simulink model "singlesource"  (Simulink 8.4)
settings: Solver=ode23tb  StartTime=0.0  StopTime=1  MaxStep=0.01  RelTol=1e-3
undefined symbols (not defined in the file): sigbuilder_block
libraries: powerlib x135, simulink x25, dsparch4 x2, powerlib_meascontrol x1
(part 1 of 2)
settings Model: Creator=Muruganandham  LastModifiedBy=SELVA
settings SolverCC: ZeroCrossControl=DisableAll

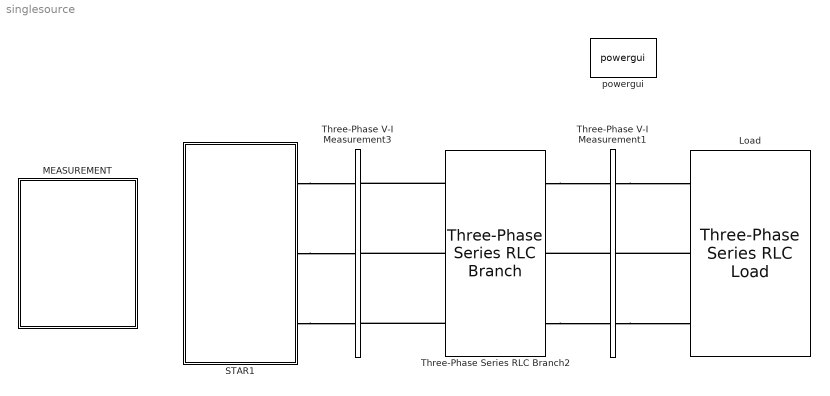
== system singlesource ==
  " Load" : powerlib/Elements/Three-Phase Series RLC Load  LConnTagsString=A|B|C  Configuration=Y (grounded)  NominalVoltage=410  NominalFrequency=50  ActivePower=5e3  InductivePower=0  CapacitivePower=0  Measurements=None  LoadType=constant Z
  MEASUREMENT : Subsystem
  STAR1 : Subsystem
  Three-Phase Series RLC Branch2 : powerlib/Elements/Three-Phase Series RLC Branch  LConnTagsString=A|B|C  RConnTagsString=A|B|C  BranchType=L  Resistance=0.0000001  Inductance=30e-3  Capacitance=3.5e-6  Measurements=None
  Three-Phase V-I Measurement1 : powerlib/Measurements/Three-Phase V-I Measurement  VoltageMeasurement=phase-to-phase  SetLabelV=on  LabelV=Vabc1  Vpu=off  VpuLL=off  CurrentMeasurement=yes  SetLabelI=on  LabelI=Iabc1  Ipu=off  Pbase=100e6  Vbase=500e3  OutputType=Complex  PhasorSimulation=off  PSBequivalent=0
  Three-Phase V-I Measurement3 : powerlib/Measurements/Three-Phase V-I Measurement  VoltageMeasurement=phase-to-phase  SetLabelV=on  LabelV=Vabc  Vpu=off  VpuLL=off  CurrentMeasurement=yes  SetLabelI=on  LabelI=Iabc  Ipu=off  Pbase=100e6  Vbase=500e3  OutputType=Complex  PhasorSimulation=off  PSBequivalent=0
  powergui : powerlib/powergui  Priority=1  SimulationMode=Discrete  SolverType=Tustin/Backward Euler (TBE)  SampleTime=5e-6  frequency=60  SPID=off  DisableSnubberDevices=off  DisableRonSwitches=off  DisableVfSwitches=off  SwTol=0  DisplayEquations=off  Interpol=off  methode=off  Ts=0  frequencyindice=0  Pbase=100e6  ErrMax=1e-4  Iterations=50  UnitsV=kV  UnitsW=MW  FunctionMessages=off  echomessages=off  HookPort=off  EnableUseOfTLC=off  x0status=blocks  RestoreLinks=warning  ResistiveCurrentMeasurement=off  Frange=[0:2:500]  Ylog=off  Xlog=on  ShowGrid=off  save=off  variable=ZData  structure=bn4  ZoomFFT=off  StartTime=0.5  cycles=1  DisplayStyle=1  fundamental=50  FreqAxis=off  MaxFrequency=1000  frequencyindicesteady=1  RmsSteady=1  display=off
  connections:
  Three-Phase V-I Measurement1/LConn1 -- " Load"/LConn1
  " Load"/LConn2 -- Three-Phase V-I Measurement1/LConn2
  Three-Phase V-I Measurement1/LConn3 -- " Load"/LConn3
  STAR1/RConn1 -- Three-Phase V-I Measurement3/RConn1
  STAR1/RConn2 -- Three-Phase V-I Measurement3/RConn2
  STAR1/RConn3 -- Three-Phase V-I Measurement3/RConn3
  Three-Phase Series RLC Branch2/LConn2 -- Three-Phase V-I Measurement3/LConn2
  Three-Phase Series RLC Branch2/LConn1 -- Three-Phase V-I Measurement3/LConn1
  Three-Phase Series RLC Branch2/LConn3 -- Three-Phase V-I Measurement3/LConn3
  Three-Phase Series RLC Branch2/RConn1 -- Three-Phase V-I Measurement1/RConn1
  Three-Phase Series RLC Branch2/RConn3 -- Three-Phase V-I Measurement1/RConn3
  Three-Phase V-I Measurement1/RConn2 -- Three-Phase Series RLC Branch2/RConn2

== system singlesource/MEASUREMENT ==
  Analog Filter Design : dsparch4/Analog Filter Design  method=Butterworth  filttype=Lowpass  N=8  Wlo=30  Whi=80  Rp=2  Rs=40
  Analog Filter Design1 : dsparch4/Analog Filter Design  method=Butterworth  filttype=Lowpass  N=8  Wlo=30  Whi=80  Rp=2  Rs=40
  Mux3 : Mux  Inputs=2
  "Power (3ph, Instantaneous)" : powerlib_meascontrol/Measurements/Power (3ph, Instantaneous)
  Scope{1,3,8..9} (4 alike) : Scope
      Scope1 settings: TimeRange=0.5  YMin=-800  YMax=800  SaveName=bn3
      Scope3 settings: TimeRange=0.5  YMin=-1000  YMax=6000  SaveName=bn2
      Scope8 settings: TimeRange=0.5  YMin=-600  YMax=800  SaveName=bn4
      Scope9 settings: YMin=-20  YMax=20
  wires:
  [Vabc] -> Scope1/1
  [Vabc1] -> "Power (3ph, Instantaneous)"/1, Scope8/1
  [Iabc1] -> "Power (3ph, Instantaneous)"/2, Scope9/1
  "Power (3ph, Instantaneous)"/1 -> Analog Filter Design/1
  "Power (3ph, Instantaneous)"/2 -> Analog Filter Design1/1
  Mux3/1 -> Scope3/1
  Analog Filter Design/1 -> Mux3/1
  Analog Filter Design1/1 -> Mux3/2

== system singlesource/STAR1 ==
  "B " : Subsystem
  DC : Subsystem
  DC1 : Subsystem
  DC2 : Subsystem
  Ground : powerlib/Elements/Ground  LConnTagsString=a
  PULSE : Subsystem  mask{fc=1000, m=1, d=0.0067}
      mask prompts: fc "Switching Frequency"; m "Modulation Index"; d "Delay"
  R : Subsystem
  Y : Subsystem
  A : PMIOPort  Tag=PMCPort  Port=1  Side=Right
  B : PMIOPort  Tag=PMCPort  Port=2  Side=Right
  C : PMIOPort  Tag=PMCPort  Port=3  Side=Right
  connections:
  Y/RConn2 -- Ground/LConn1 -- "B "/RConn2 -- R/RConn2
  DC/RConn1 -- R/LConn1
  DC/RConn3 -- R/LConn3
  DC/RConn4 -- R/LConn4
  DC/RConn9 -- R/LConn9
  DC/RConn2 -- R/LConn2
  DC/RConn5 -- R/LConn5
  DC/RConn7 -- R/LConn7
  DC/RConn6 -- R/LConn6
  DC/RConn8 -- R/LConn8
  DC/RConn10 -- R/LConn10
  DC1/RConn1 -- Y/LConn1
  DC1/RConn2 -- Y/LConn2
  DC1/RConn3 -- Y/LConn3
  DC1/RConn4 -- Y/LConn4
  DC1/RConn5 -- Y/LConn5
  DC1/RConn6 -- Y/LConn6
  DC1/RConn7 -- Y/LConn7
  DC1/RConn8 -- Y/LConn8
  DC1/RConn9 -- Y/LConn9
  DC1/RConn10 -- Y/LConn10
  DC2/RConn1 -- "B "/LConn1
  DC2/RConn2 -- "B "/LConn2
  DC2/RConn3 -- "B "/LConn3
  DC2/RConn4 -- "B "/LConn4
  DC2/RConn5 -- "B "/LConn5
  DC2/RConn6 -- "B "/LConn6
  DC2/RConn7 -- "B "/LConn7
  DC2/RConn8 -- "B "/LConn8
  DC2/RConn9 -- "B "/LConn9
  DC2/RConn10 -- "B "/LConn10
  A/RConn1 -- R/RConn1
  B/RConn1 -- Y/RConn1
  C/RConn1 -- "B "/RConn1

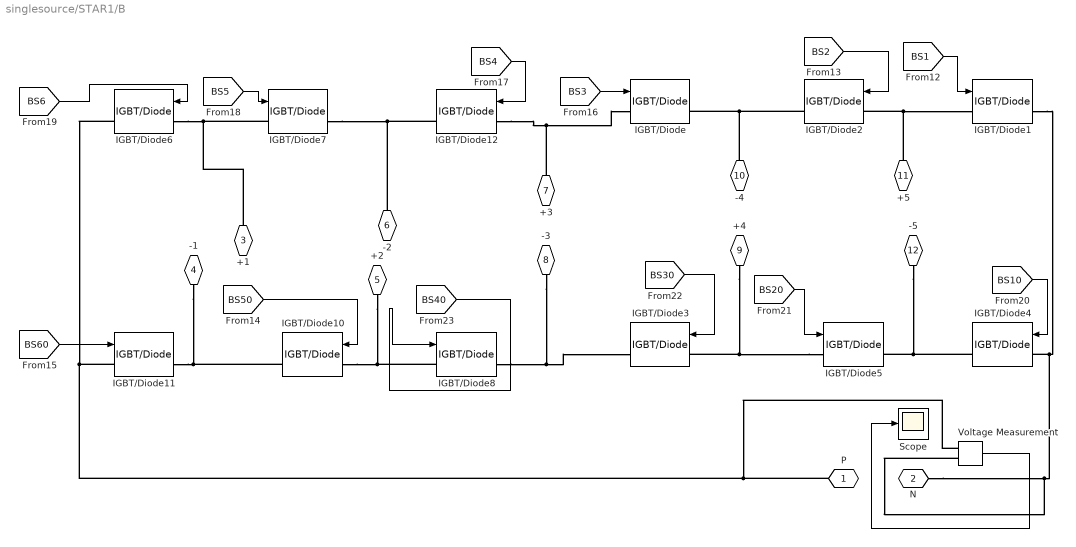
== system singlesource/STAR1/B  ==
  IGBT/Diode{,1..8,10..12} (12 alike) : powerlib/Power Electronics/IGBT//Diode  Ron=1e-3  Rs=1e5  Cs=inf  Measurements=on
  Scope : Scope
  Voltage Measurement : powerlib/Measurements/Voltage Measurement  PhasorSimulation=off  OutputType=Complex  PSBequivalent=0
  P : PMIOPort  Tag=PMCPort  Port=1  Side=Right
  N : PMIOPort  Tag=PMCPort  Port=2  Side=Right
  +1 : PMIOPort  Tag=PMCPort  Port=3  Side=Left
  -1 : PMIOPort  Tag=PMCPort  Port=4  Side=Left
  +2 : PMIOPort  Tag=PMCPort  Port=5  Side=Left
  -2 : PMIOPort  Tag=PMCPort  Port=6  Side=Left
  +3 : PMIOPort  Tag=PMCPort  Port=7  Side=Left
  -3 : PMIOPort  Tag=PMCPort  Port=8  Side=Left
  +4 : PMIOPort  Tag=PMCPort  Port=9  Side=Left
  -4 : PMIOPort  Tag=PMCPort  Port=10  Side=Left
  +5 : PMIOPort  Tag=PMCPort  Port=11  Side=Left
  -5 : PMIOPort  Tag=PMCPort  Port=12  Side=Left
  wires:
  [BS10] -> IGBT/Diode4/1
  [BS2] -> IGBT/Diode2/1
  [BS20] -> IGBT/Diode5/1
  [BS3] -> IGBT/Diode/1
  [BS30] -> IGBT/Diode3/1
  [BS40] -> IGBT/Diode8/1
  [BS6] -> IGBT/Diode6/1
  [BS4] -> IGBT/Diode12/1
  [BS5] -> IGBT/Diode7/1
  [BS50] -> IGBT/Diode10/1
  [BS60] -> IGBT/Diode11/1
  Voltage Measurement/1 -> Scope/1
  [BS1] -> IGBT/Diode1/1
  connections:
  IGBT/Diode2/RConn1 -- -4/RConn1 -- IGBT/Diode/RConn1
  IGBT/Diode2/LConn1 -- IGBT/Diode1/LConn1 -- +5/RConn1
  IGBT/Diode5/LConn1 -- +4/RConn1 -- IGBT/Diode3/LConn1
  IGBT/Diode4/RConn1 -- -5/RConn1 -- IGBT/Diode5/RConn1
  IGBT/Diode4/LConn1 -- IGBT/Diode1/RConn1 -- N/RConn1 -- Voltage Measurement/LConn2
  IGBT/Diode7/LConn1 -- +1/RConn1 -- IGBT/Diode6/LConn1
  IGBT/Diode12/RConn1 -- IGBT/Diode7/RConn1 -- -2/RConn1
  IGBT/Diode10/RConn1 -- IGBT/Diode11/RConn1 -- -1/RConn1
  IGBT/Diode8/LConn1 -- IGBT/Diode10/LConn1 -- +2/RConn1
  IGBT/Diode12/LConn1 -- IGBT/Diode/LConn1 -- +3/RConn1
  IGBT/Diode8/RConn1 -- IGBT/Diode3/RConn1 -- -3/RConn1
  IGBT/Diode6/RConn1 -- IGBT/Diode11/LConn1 -- P/RConn1 -- Voltage Measurement/LConn1

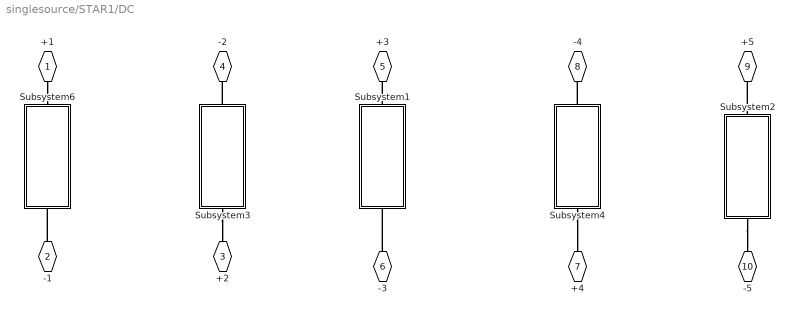
== system singlesource/STAR1/DC ==
  Subsystem1 : Subsystem
  Subsystem2 : Subsystem
  Subsystem3 : Subsystem
  Subsystem4 : Subsystem
  Subsystem6 : Subsystem
  +1 : PMIOPort  Tag=PMCPort  Port=1  Side=Right
  -1 : PMIOPort  Tag=PMCPort  Port=2  Side=Right
  +2 : PMIOPort  Tag=PMCPort  Port=3  Side=Right
  -2 : PMIOPort  Tag=PMCPort  Port=4  Side=Right
  +3 : PMIOPort  Tag=PMCPort  Port=5  Side=Right
  -3 : PMIOPort  Tag=PMCPort  Port=6  Side=Right
  +4 : PMIOPort  Tag=PMCPort  Port=7  Side=Right
  -4 : PMIOPort  Tag=PMCPort  Port=8  Side=Right
  +5 : PMIOPort  Tag=PMCPort  Port=9  Side=Right
  -5 : PMIOPort  Tag=PMCPort  Port=10  Side=Right
  connections:
  -1/RConn1 -- Subsystem6/RConn1
  +1/RConn1 -- Subsystem6/LConn1
  -3/RConn1 -- Subsystem1/RConn1
  Subsystem4/LConn1 -- +4/RConn1
  Subsystem2/RConn1 -- -5/RConn1
  Subsystem1/LConn1 -- +3/RConn1
  Subsystem2/LConn1 -- +5/RConn1
  Subsystem4/RConn1 -- -4/RConn1
  Subsystem3/RConn1 -- -2/RConn1
  Subsystem3/LConn1 -- +2/RConn1

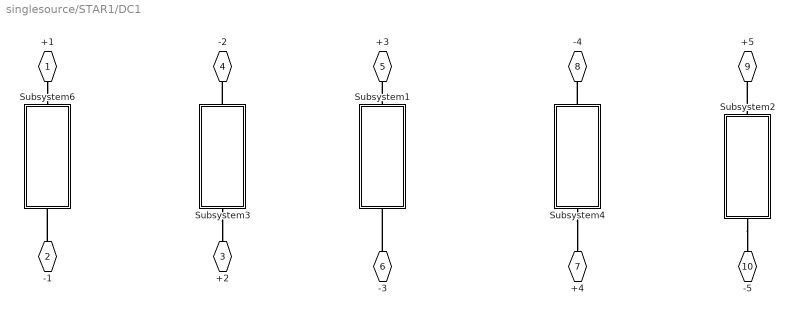
== system singlesource/STAR1/DC1 ==
  Subsystem1 : Subsystem
  Subsystem2 : Subsystem
  Subsystem3 : Subsystem
  Subsystem4 : Subsystem
  Subsystem6 : Subsystem
  +1 : PMIOPort  Tag=PMCPort  Port=1  Side=Right
  -1 : PMIOPort  Tag=PMCPort  Port=2  Side=Right
  +2 : PMIOPort  Tag=PMCPort  Port=3  Side=Right
  -2 : PMIOPort  Tag=PMCPort  Port=4  Side=Right
  +3 : PMIOPort  Tag=PMCPort  Port=5  Side=Right
  -3 : PMIOPort  Tag=PMCPort  Port=6  Side=Right
  +4 : PMIOPort  Tag=PMCPort  Port=7  Side=Right
  -4 : PMIOPort  Tag=PMCPort  Port=8  Side=Right
  +5 : PMIOPort  Tag=PMCPort  Port=9  Side=Right
  -5 : PMIOPort  Tag=PMCPort  Port=10  Side=Right
  connections:
  Subsystem3/LConn1 -- +2/RConn1
  Subsystem3/RConn1 -- -2/RConn1
  Subsystem4/RConn1 -- -4/RConn1
  Subsystem2/LConn1 -- +5/RConn1
  Subsystem1/LConn1 -- +3/RConn1
  Subsystem2/RConn1 -- -5/RConn1
  Subsystem4/LConn1 -- +4/RConn1
  -3/RConn1 -- Subsystem1/RConn1
  +1/RConn1 -- Subsystem6/LConn1
  -1/RConn1 -- Subsystem6/RConn1

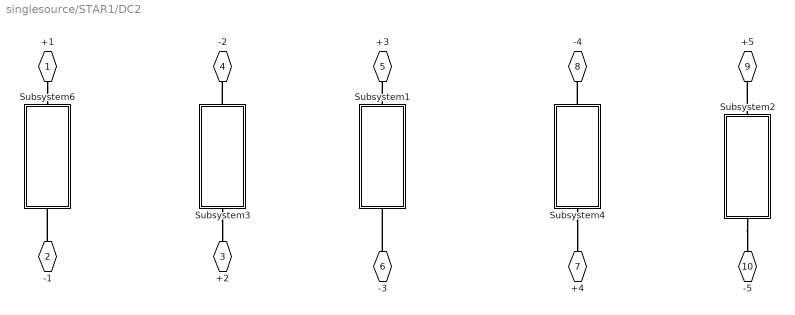
== system singlesource/STAR1/DC2 ==
  Subsystem1 : Subsystem
  Subsystem2 : Subsystem
  Subsystem3 : Subsystem
  Subsystem4 : Subsystem
  Subsystem6 : Subsystem
  +1 : PMIOPort  Tag=PMCPort  Port=1  Side=Right
  -1 : PMIOPort  Tag=PMCPort  Port=2  Side=Right
  +2 : PMIOPort  Tag=PMCPort  Port=3  Side=Right
  -2 : PMIOPort  Tag=PMCPort  Port=4  Side=Right
  +3 : PMIOPort  Tag=PMCPort  Port=5  Side=Right
  -3 : PMIOPort  Tag=PMCPort  Port=6  Side=Right
  +4 : PMIOPort  Tag=PMCPort  Port=7  Side=Right
  -4 : PMIOPort  Tag=PMCPort  Port=8  Side=Right
  +5 : PMIOPort  Tag=PMCPort  Port=9  Side=Right
  -5 : PMIOPort  Tag=PMCPort  Port=10  Side=Right
  connections:
  -1/RConn1 -- Subsystem6/RConn1
  +1/RConn1 -- Subsystem6/LConn1
  -3/RConn1 -- Subsystem1/RConn1
  Subsystem4/LConn1 -- +4/RConn1
  Subsystem2/RConn1 -- -5/RConn1
  Subsystem1/LConn1 -- +3/RConn1
  Subsystem2/LConn1 -- +5/RConn1
  Subsystem4/RConn1 -- -4/RConn1
  Subsystem3/RConn1 -- -2/RConn1
  Subsystem3/LConn1 -- +2/RConn1

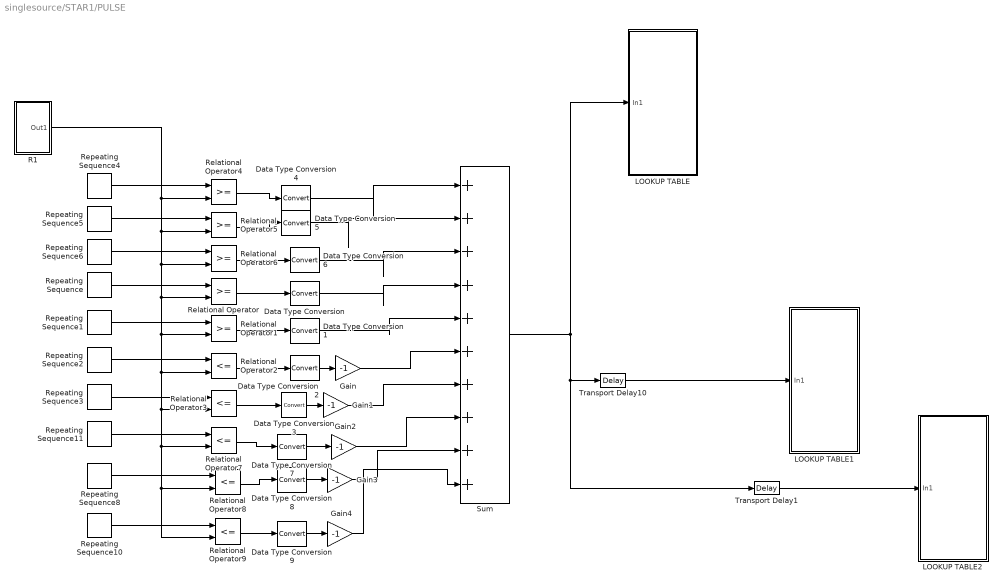
== system singlesource/STAR1/PULSE ==
  Data Type Conversion{,1..9} (10 alike) : DataTypeConversion
  Gain{,1..4} (5 alike) : Gain  Gain=-1
  LOOKUP TABLE : Subsystem
  LOOKUP TABLE1 : Subsystem
  LOOKUP TABLE2 : Subsystem
  R1 : Subsystem
  Relational Operator{,1,4..6} (5 alike) : RelationalOperator  OutDataTypeStr=boolean
  Relational Operator{2..3,7..9} (5 alike) : RelationalOperator  Operator=<=  OutDataTypeStr=boolean
  Repeating Sequence : simulink/Sources/Repeating Sequence  rep_seq_t="[0 (1/fc)/2  (1/fc)]"  rep_seq_y=[2 1 2]
  Repeating Sequence1 : simulink/Sources/Repeating Sequence  rep_seq_t="[0 (1/fc)/2  (1/fc)]"  rep_seq_y=[1 0 1]
  Repeating Sequence10 : simulink/Sources/Repeating Sequence  rep_seq_t="[0 (0.1/fc)/2  (0.1/fc)]"  rep_seq_y=[-5 -4 -5]
  Repeating Sequence11 : simulink/Sources/Repeating Sequence  rep_seq_t="[0 (1/fc)/2  (1/fc)]"  rep_seq_y=[-3 -2 -3]
  Repeating Sequence2 : simulink/Sources/Repeating Sequence  rep_seq_t="[0 (1/fc)/2  (1/fc)]"  rep_seq_y=[-1 0 -1]
  Repeating Sequence3 : simulink/Sources/Repeating Sequence  rep_seq_t="[0 (1/fc)/2  (1/fc)]"  rep_seq_y=[-2 -1 -2]
  Repeating Sequence4 : simulink/Sources/Repeating Sequence  rep_seq_t="[0 (0.1/fc)/2  (0.1/fc)]"  rep_seq_y=[4 5 4]
  Repeating Sequence5 : simulink/Sources/Repeating Sequence  rep_seq_t="[0 (1/fc)/2  (1/fc)]"  rep_seq_y=[4 3 4]
  Repeating Sequence6 : simulink/Sources/Repeating Sequence  rep_seq_t="[0 (1/fc)/2  (1/fc)]"  rep_seq_y=[3 2 3]
  Repeating Sequence8 : simulink/Sources/Repeating Sequence  rep_seq_t="[0 (1/fc)/2  (1/fc)]"  rep_seq_y=[-4 -3 -4]
  Sum : Sum  Inputs=|++++++++++
  Transport Delay1 : TransportDelay  DelayTime=2*d
  Transport Delay10 : TransportDelay  DelayTime=d
  wires:
  Data Type Conversion3/1 -> Gain1/1
  Data Type Conversion2/1 -> Gain/1
  Relational Operator3/1 -> Data Type Conversion3/1
  Relational Operator2/1 -> Data Type Conversion2/1
  Repeating Sequence3/1 -> Relational Operator3/1
  Repeating Sequence2/1 -> Relational Operator2/1
  Repeating Sequence1/1 -> Relational Operator1/1
  Repeating Sequence/1 -> Relational Operator/1
  Relational Operator1/1 -> Data Type Conversion1/1
  Relational Operator/1 -> Data Type Conversion/1
  Repeating Sequence6/1 -> Relational Operator6/1
  Repeating Sequence5/1 -> Relational Operator5/1
  Repeating Sequence4/1 -> Relational Operator4/1
  Relational Operator6/1 -> Data Type Conversion6/1
  Relational Operator5/1 -> Data Type Conversion5/1
  Relational Operator4/1 -> Data Type Conversion4/1
  Repeating Sequence8/1 -> Relational Operator8/1
  Repeating Sequence11/1 -> Relational Operator7/1
  Relational Operator9/1 -> Data Type Conversion9/1
  Relational Operator8/1 -> Data Type Conversion8/1
  Relational Operator7/1 -> Data Type Conversion7/1
  Data Type Conversion9/1 -> Gain4/1
  Data Type Conversion8/1 -> Gain3/1
  Data Type Conversion7/1 -> Gain2/1
  Repeating Sequence10/1 -> Relational Operator9/1
  Data Type Conversion4/1 -> Sum/1
  Data Type Conversion5/1 -> Sum/2
  Data Type Conversion6/1 -> Sum/3
  Data Type Conversion/1 -> Sum/4
  Data Type Conversion1/1 -> Sum/5
  Gain/1 -> Sum/6
  Gain1/1 -> Sum/7
  Gain2/1 -> Sum/8
  Gain3/1 -> Sum/9
  Gain4/1 -> Sum/10
  Transport Delay10/1 -> LOOKUP TABLE1/1(In1)
  Sum/1 -> LOOKUP TABLE/1(In1), Transport Delay1/1, Transport Delay10/1
  Transport Delay1/1 -> LOOKUP TABLE2/1(In1)
  R1/1(Out1) -> Relational Operator4/2, Relational Operator5/2, Relational Operator6/2, Relational Operator1/2, Relational Operator2/2, Relational Operator3/2, Relational Operator7/2, Relational Operator8/2, Relational Operator9/2, Relational Operator/2

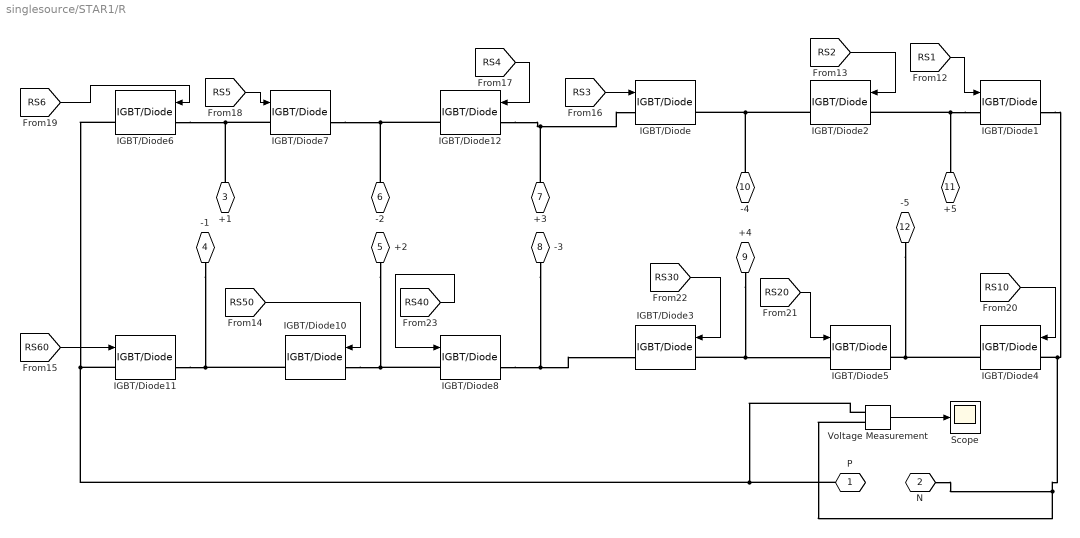
== system singlesource/STAR1/R ==
  IGBT/Diode{,1..8,10..12} (12 alike) : powerlib/Power Electronics/IGBT//Diode  Ron=1e-3  Rs=1e5  Cs=inf  Measurements=on
  Scope : Scope
  Voltage Measurement : powerlib/Measurements/Voltage Measurement  PhasorSimulation=off  OutputType=Complex  PSBequivalent=0
  P : PMIOPort  Tag=PMCPort  Port=1  Side=Right
  N : PMIOPort  Tag=PMCPort  Port=2  Side=Right
  +1 : PMIOPort  Tag=PMCPort  Port=3  Side=Left
  -1 : PMIOPort  Tag=PMCPort  Port=4  Side=Left
  +2 : PMIOPort  Tag=PMCPort  Port=5  Side=Left
  -2 : PMIOPort  Tag=PMCPort  Port=6  Side=Left
  +3 : PMIOPort  Tag=PMCPort  Port=7  Side=Left
  -3 : PMIOPort  Tag=PMCPort  Port=8  Side=Left
  +4 : PMIOPort  Tag=PMCPort  Port=9  Side=Left
  -4 : PMIOPort  Tag=PMCPort  Port=10  Side=Left
  +5 : PMIOPort  Tag=PMCPort  Port=11  Side=Left
  -5 : PMIOPort  Tag=PMCPort  Port=12  Side=Left
  wires:
  [RS10] -> IGBT/Diode4/1
  [RS2] -> IGBT/Diode2/1
  [RS20] -> IGBT/Diode5/1
  [RS3] -> IGBT/Diode/1
  [RS30] -> IGBT/Diode3/1
  [RS40] -> IGBT/Diode8/1
  [RS6] -> IGBT/Diode6/1
  [RS4] -> IGBT/Diode12/1
  [RS5] -> IGBT/Diode7/1
  [RS50] -> IGBT/Diode10/1
  [RS60] -> IGBT/Diode11/1
  Voltage Measurement/1 -> Scope/1
  [RS1] -> IGBT/Diode1/1
  connections:
  IGBT/Diode2/RConn1 -- -4/RConn1 -- IGBT/Diode/RConn1
  IGBT/Diode1/LConn1 -- IGBT/Diode2/LConn1 -- +5/RConn1
  +4/RConn1 -- IGBT/Diode5/LConn1 -- IGBT/Diode3/LConn1
  IGBT/Diode4/RConn1 -- -5/RConn1 -- IGBT/Diode5/RConn1
  IGBT/Diode4/LConn1 -- Voltage Measurement/LConn2 -- N/RConn1 -- IGBT/Diode1/RConn1
  IGBT/Diode7/LConn1 -- IGBT/Diode6/LConn1 -- +1/RConn1
  IGBT/Diode12/RConn1 -- -2/RConn1 -- IGBT/Diode7/RConn1
  IGBT/Diode10/RConn1 -- IGBT/Diode11/RConn1 -- -1/RConn1
  IGBT/Diode8/LConn1 -- +2/RConn1 -- IGBT/Diode10/LConn1
  IGBT/Diode12/LConn1 -- IGBT/Diode/LConn1 -- +3/RConn1
  IGBT/Diode8/RConn1 -- IGBT/Diode3/RConn1 -- -3/RConn1
  IGBT/Diode6/RConn1 -- Voltage Measurement/LConn1 -- P/RConn1 -- IGBT/Diode11/LConn1

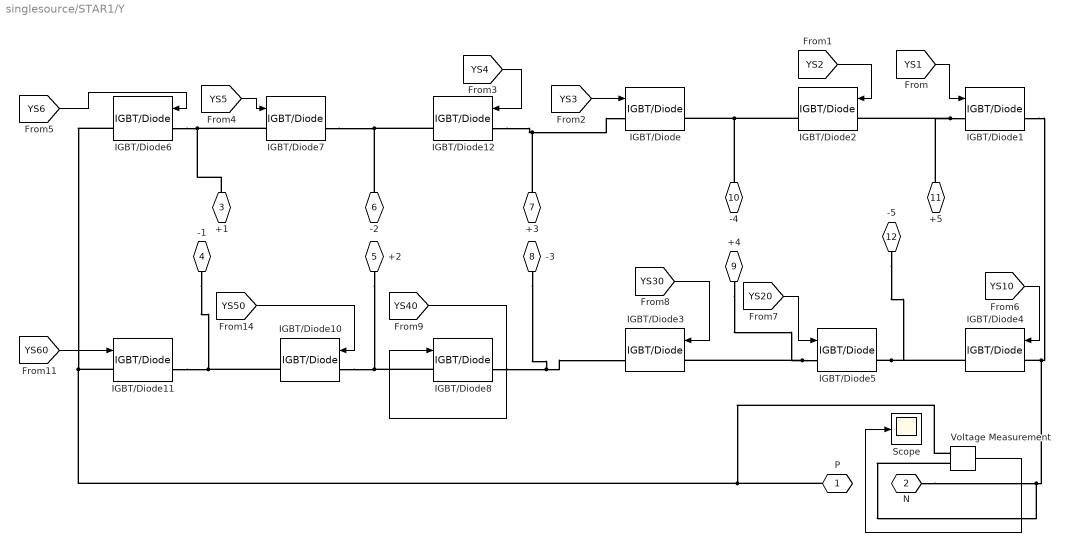
== system singlesource/STAR1/Y ==
  IGBT/Diode{,1..8,10..12} (12 alike) : powerlib/Power Electronics/IGBT//Diode  Ron=1e-3  Rs=1e5  Cs=inf  Measurements=on
  Scope : Scope
  Voltage Measurement : powerlib/Measurements/Voltage Measurement  PhasorSimulation=off  OutputType=Complex  PSBequivalent=0
  P : PMIOPort  Tag=PMCPort  Port=1  Side=Right
  N : PMIOPort  Tag=PMCPort  Port=2  Side=Right
  +1 : PMIOPort  Tag=PMCPort  Port=3  Side=Left
  -1 : PMIOPort  Tag=PMCPort  Port=4  Side=Left
  +2 : PMIOPort  Tag=PMCPort  Port=5  Side=Left
  -2 : PMIOPort  Tag=PMCPort  Port=6  Side=Left
  +3 : PMIOPort  Tag=PMCPort  Port=7  Side=Left
  -3 : PMIOPort  Tag=PMCPort  Port=8  Side=Left
  +4 : PMIOPort  Tag=PMCPort  Port=9  Side=Left
  -4 : PMIOPort  Tag=PMCPort  Port=10  Side=Left
  +5 : PMIOPort  Tag=PMCPort  Port=11  Side=Left
  -5 : PMIOPort  Tag=PMCPort  Port=12  Side=Left
  wires:
  [YS1] -> IGBT/Diode1/1
  Voltage Measurement/1 -> Scope/1
  [YS60] -> IGBT/Diode11/1
  [YS50] -> IGBT/Diode10/1
  [YS5] -> IGBT/Diode7/1
  [YS4] -> IGBT/Diode12/1
  [YS6] -> IGBT/Diode6/1
  [YS40] -> IGBT/Diode8/1
  [YS30] -> IGBT/Diode3/1
  [YS3] -> IGBT/Diode/1
  [YS20] -> IGBT/Diode5/1
  [YS2] -> IGBT/Diode2/1
  [YS10] -> IGBT/Diode4/1
  connections:
  Voltage Measurement/LConn1 -- P/RConn1 -- IGBT/Diode11/LConn1 -- IGBT/Diode6/RConn1
  IGBT/Diode8/RConn1 -- -3/RConn1 -- IGBT/Diode3/RConn1
  IGBT/Diode12/LConn1 -- +3/RConn1 -- IGBT/Diode/LConn1
  IGBT/Diode10/LConn1 -- IGBT/Diode8/LConn1 -- +2/RConn1
  IGBT/Diode11/RConn1 -- IGBT/Diode10/RConn1 -- -1/RConn1
  IGBT/Diode7/RConn1 -- IGBT/Diode12/RConn1 -- -2/RConn1
  IGBT/Diode6/LConn1 -- IGBT/Diode7/LConn1 -- +1/RConn1
  Voltage Measurement/LConn2 -- N/RConn1 -- IGBT/Diode1/RConn1 -- IGBT/Diode4/LConn1
  IGBT/Diode5/RConn1 -- IGBT/Diode4/RConn1 -- -5/RConn1
  IGBT/Diode5/LConn1 -- IGBT/Diode3/LConn1 -- +4/RConn1
  IGBT/Diode1/LConn1 -- IGBT/Diode2/LConn1 -- +5/RConn1
  IGBT/Diode2/RConn1 -- IGBT/Diode/RConn1 -- -4/RConn1

== system singlesource/STAR1/DC/Subsystem1 ==
  DC Voltage Source : powerlib/Electrical Sources/DC Voltage Source  Amplitude=24  Measurements=None
  PV Boost Converter1 : Subsystem
  + : PMIOPort  Port=1  Side=Left
  - : PMIOPort  Port=2  Side=Right
  connections:
  DC Voltage Source/LConn1 -- PV Boost Converter1/LConn2
  DC Voltage Source/RConn1 -- PV Boost Converter1/LConn1
  PV Boost Converter1/RConn2 -- -/RConn1
  PV Boost Converter1/RConn1 -- +/RConn1

== system singlesource/STAR1/DC/Subsystem2 ==
  DC Voltage Source : powerlib/Electrical Sources/DC Voltage Source  Amplitude=24  Measurements=None
  PV Boost Converter1 : Subsystem
  + : PMIOPort  Port=1  Side=Left
  - : PMIOPort  Port=2  Side=Right
  connections:
  PV Boost Converter1/RConn1 -- +/RConn1
  PV Boost Converter1/RConn2 -- -/RConn1
  DC Voltage Source/RConn1 -- PV Boost Converter1/LConn1
  DC Voltage Source/LConn1 -- PV Boost Converter1/LConn2

== system singlesource/STAR1/DC/Subsystem3 ==
  DC Voltage Source : powerlib/Electrical Sources/DC Voltage Source  Amplitude=24  Measurements=None
  PV Boost Converter1 : Subsystem
  + : PMIOPort  Port=1  Side=Left
  - : PMIOPort  Port=2  Side=Right
  connections:
  PV Boost Converter1/RConn1 -- +/RConn1
  PV Boost Converter1/RConn2 -- -/RConn1
  DC Voltage Source/RConn1 -- PV Boost Converter1/LConn1
  DC Voltage Source/LConn1 -- PV Boost Converter1/LConn2

== system singlesource/STAR1/DC/Subsystem4 ==
  DC Voltage Source : powerlib/Electrical Sources/DC Voltage Source  Amplitude=24  Measurements=None
  PV Boost Converter1 : Subsystem
  + : PMIOPort  Port=1  Side=Left
  - : PMIOPort  Port=2  Side=Right
  connections:
  DC Voltage Source/LConn1 -- PV Boost Converter1/LConn2
  DC Voltage Source/RConn1 -- PV Boost Converter1/LConn1
  PV Boost Converter1/RConn2 -- -/RConn1
  PV Boost Converter1/RConn1 -- +/RConn1

== system singlesource/STAR1/DC/Subsystem6 ==
  DC Voltage Source : powerlib/Electrical Sources/DC Voltage Source  Amplitude=24  Measurements=None
  PV Boost Converter1 : Subsystem
  + : PMIOPort  Port=1  Side=Left
  - : PMIOPort  Port=2  Side=Right
  connections:
  PV Boost Converter1/RConn1 -- +/RConn1
  PV Boost Converter1/RConn2 -- -/RConn1
  DC Voltage Source/RConn1 -- PV Boost Converter1/LConn1
  DC Voltage Source/LConn1 -- PV Boost Converter1/LConn2

== system singlesource/STAR1/DC1/Subsystem1 ==
  DC Voltage Source : powerlib/Electrical Sources/DC Voltage Source  Amplitude=24  Measurements=None
  PV Boost Converter1 : Subsystem
  + : PMIOPort  Port=1  Side=Left
  - : PMIOPort  Port=2  Side=Right
  connections:
  PV Boost Converter1/RConn1 -- +/RConn1
  PV Boost Converter1/RConn2 -- -/RConn1
  DC Voltage Source/RConn1 -- PV Boost Converter1/LConn1
  DC Voltage Source/LConn1 -- PV Boost Converter1/LConn2

== system singlesource/STAR1/DC1/Subsystem2 ==
  DC Voltage Source : powerlib/Electrical Sources/DC Voltage Source  Amplitude=24  Measurements=None
  PV Boost Converter1 : Subsystem
  + : PMIOPort  Port=1  Side=Left
  - : PMIOPort  Port=2  Side=Right
  connections:
  DC Voltage Source/LConn1 -- PV Boost Converter1/LConn2
  DC Voltage Source/RConn1 -- PV Boost Converter1/LConn1
  PV Boost Converter1/RConn2 -- -/RConn1
  PV Boost Converter1/RConn1 -- +/RConn1

== system singlesource/STAR1/DC1/Subsystem3 ==
  DC Voltage Source : powerlib/Electrical Sources/DC Voltage Source  Amplitude=24  Measurements=None
  PV Boost Converter1 : Subsystem
  + : PMIOPort  Port=1  Side=Left
  - : PMIOPort  Port=2  Side=Right
  connections:
  DC Voltage Source/LConn1 -- PV Boost Converter1/LConn2
  DC Voltage Source/RConn1 -- PV Boost Converter1/LConn1
  PV Boost Converter1/RConn2 -- -/RConn1
  PV Boost Converter1/RConn1 -- +/RConn1

== system singlesource/STAR1/DC1/Subsystem4 ==
  DC Voltage Source : powerlib/Electrical Sources/DC Voltage Source  Amplitude=24  Measurements=None
  PV Boost Converter1 : Subsystem
  + : PMIOPort  Port=1  Side=Left
  - : PMIOPort  Port=2  Side=Right
  connections:
  PV Boost Converter1/RConn1 -- +/RConn1
  PV Boost Converter1/RConn2 -- -/RConn1
  DC Voltage Source/RConn1 -- PV Boost Converter1/LConn1
  DC Voltage Source/LConn1 -- PV Boost Converter1/LConn2

== system singlesource/STAR1/DC1/Subsystem6 ==
  DC Voltage Source : powerlib/Electrical Sources/DC Voltage Source  Amplitude=24  Measurements=None
  PV Boost Converter1 : Subsystem
  + : PMIOPort  Port=1  Side=Left
  - : PMIOPort  Port=2  Side=Right
  connections:
  DC Voltage Source/LConn1 -- PV Boost Converter1/LConn2
  DC Voltage Source/RConn1 -- PV Boost Converter1/LConn1
  PV Boost Converter1/RConn2 -- -/RConn1
  PV Boost Converter1/RConn1 -- +/RConn1

== system singlesource/STAR1/DC2/Subsystem1 ==
  DC Voltage Source : powerlib/Electrical Sources/DC Voltage Source  Amplitude=24  Measurements=None
  PV Boost Converter1 : Subsystem
  + : PMIOPort  Port=1  Side=Left
  - : PMIOPort  Port=2  Side=Right
  connections:
  DC Voltage Source/LConn1 -- PV Boost Converter1/LConn2
  DC Voltage Source/RConn1 -- PV Boost Converter1/LConn1
  PV Boost Converter1/RConn2 -- -/RConn1
  PV Boost Converter1/RConn1 -- +/RConn1

== system singlesource/STAR1/DC2/Subsystem2 ==
  DC Voltage Source : powerlib/Electrical Sources/DC Voltage Source  Amplitude=24  Measurements=None
  PV Boost Converter1 : Subsystem
  + : PMIOPort  Port=1  Side=Left
  - : PMIOPort  Port=2  Side=Right
  connections:
  PV Boost Converter1/RConn1 -- +/RConn1
  PV Boost Converter1/RConn2 -- -/RConn1
  DC Voltage Source/RConn1 -- PV Boost Converter1/LConn1
  DC Voltage Source/LConn1 -- PV Boost Converter1/LConn2

== system singlesource/STAR1/DC2/Subsystem3 ==
  DC Voltage Source : powerlib/Electrical Sources/DC Voltage Source  Amplitude=24  Measurements=None
  PV Boost Converter1 : Subsystem
  + : PMIOPort  Port=1  Side=Left
  - : PMIOPort  Port=2  Side=Right
  connections:
  PV Boost Converter1/RConn1 -- +/RConn1
  PV Boost Converter1/RConn2 -- -/RConn1
  DC Voltage Source/RConn1 -- PV Boost Converter1/LConn1
  DC Voltage Source/LConn1 -- PV Boost Converter1/LConn2

== system singlesource/STAR1/DC2/Subsystem4 ==
  DC Voltage Source : powerlib/Electrical Sources/DC Voltage Source  Amplitude=24  Measurements=None
  PV Boost Converter1 : Subsystem
  + : PMIOPort  Port=1  Side=Left
  - : PMIOPort  Port=2  Side=Right
  connections:
  DC Voltage Source/LConn1 -- PV Boost Converter1/LConn2
  DC Voltage Source/RConn1 -- PV Boost Converter1/LConn1
  PV Boost Converter1/RConn2 -- -/RConn1
  PV Boost Converter1/RConn1 -- +/RConn1

== system singlesource/STAR1/DC2/Subsystem6 ==
  DC Voltage Source : powerlib/Electrical Sources/DC Voltage Source  Amplitude=24  Measurements=None
  PV Boost Converter1 : Subsystem
  + : PMIOPort  Port=1  Side=Left
  - : PMIOPort  Port=2  Side=Right
  connections:
  PV Boost Converter1/RConn1 -- +/RConn1
  PV Boost Converter1/RConn2 -- -/RConn1
  DC Voltage Source/RConn1 -- PV Boost Converter1/LConn1
  DC Voltage Source/LConn1 -- PV Boost Converter1/LConn2

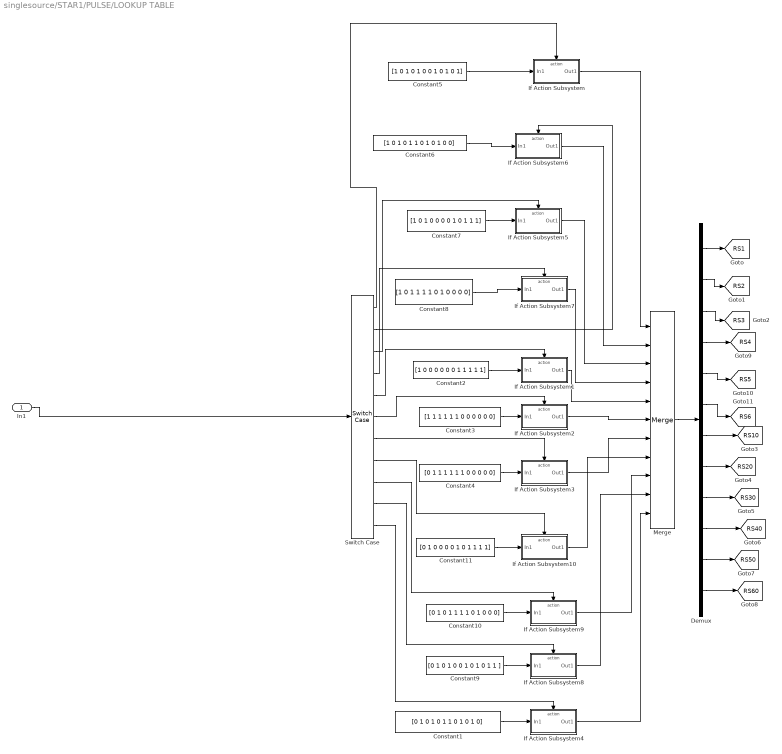
== system singlesource/STAR1/PULSE/LOOKUP TABLE ==
  In1 : Inport
  Constant1 : Constant  Value=[0 1 0 1 0 1 1 0 1 0 1 0]
  Constant10 : Constant  Value=[0 1 0 1 1 1 1 0 1 0 0 0]
  Constant11 : Constant  Value=[0 1 0 0 0 0 1 0 1 1 1 1]
  Constant2 : Constant  Value=[1 0 0 0 0 0 0 1 1 1 1 1]
  Constant3 : Constant  Value=[1 1 1 1 1 1 0 0 0 0 0 0]
  Constant4 : Constant  Value=[0 1 1 1 1 1 1 0 0 0 0 0]
  Constant5 : Constant  Value=[1 0 1 0 1 0 0 1 0 1 0 1]
  Constant6 : Constant  Value=[1 0 1 0 1 1 0 1 0 1 0 0]
  Constant7 : Constant  Value=[1 0 1 0 0 0 0 1 0 1 1 1]
  Constant8 : Constant  Value=[1 0 1 1 1 1 0 1 0 0 0 0]
  Constant9 : Constant  Value=[0 1 0 1 0 0 1 0 1 0 1 1 ]
  Demux : Demux  Outputs=12
  If Action Subsystem : Subsystem  TreatAsAtomicUnit=on
  If Action Subsystem1 : Subsystem  TreatAsAtomicUnit=on
  If Action Subsystem10 : Subsystem  TreatAsAtomicUnit=on
  If Action Subsystem2 : Subsystem  TreatAsAtomicUnit=on
  If Action Subsystem3 : Subsystem  TreatAsAtomicUnit=on
  If Action Subsystem4 : Subsystem  TreatAsAtomicUnit=on
  If Action Subsystem5 : Subsystem  TreatAsAtomicUnit=on
  If Action Subsystem6 : Subsystem  TreatAsAtomicUnit=on
  If Action Subsystem7 : Subsystem  TreatAsAtomicUnit=on
  If Action Subsystem8 : Subsystem  TreatAsAtomicUnit=on
  If Action Subsystem9 : Subsystem  TreatAsAtomicUnit=on
  Merge : Merge  Inputs=11
  Switch Case : SwitchCase  CaseConditions={-5 -4 -3 -2 -1 0 1 2 3 4 5}  ShowDefaultCase=off
  tag scope: RS10=global, RS1=global, RS20=global, RS2=global, RS30=global, RS3=global, RS40=global, RS4=global, RS50=global, RS5=global, RS60=global, RS6=global
  wires:
  Merge/1 -> Demux/1
  If Action Subsystem/1(Out1) -> Merge/1
  Constant4/1 -> If Action Subsystem3/1(In1)
  Constant3/1 -> If Action Subsystem2/1(In1)
  Constant2/1 -> If Action Subsystem1/1(In1)
  Switch Case/6 -> If Action Subsystem2/Action
  If Action Subsystem6/1(Out1) -> Merge/2
  If Action Subsystem5/1(Out1) -> Merge/3
  If Action Subsystem7/1(Out1) -> Merge/4
  If Action Subsystem1/1(Out1) -> Merge/5
  If Action Subsystem2/1(Out1) -> Merge/6
  If Action Subsystem3/1(Out1) -> Merge/7
  Constant9/1 -> If Action Subsystem8/1(In1)
  Constant10/1 -> If Action Subsystem9/1(In1)
  Constant11/1 -> If Action Subsystem10/1(In1)
  Switch Case/11 -> If Action Subsystem4/Action
  If Action Subsystem4/1(Out1) -> Merge/11
  Switch Case/10 -> If Action Subsystem8/Action
  Switch Case/9 -> If Action Subsystem9/Action
  Switch Case/8 -> If Action Subsystem10/Action
  Switch Case/7 -> If Action Subsystem3/Action
  Switch Case/5 -> If Action Subsystem1/Action
  Switch Case/4 -> If Action Subsystem7/Action
  Switch Case/3 -> If Action Subsystem5/Action
  Switch Case/2 -> If Action Subsystem6/Action
  Switch Case/1 -> If Action Subsystem/Action
  Constant6/1 -> If Action Subsystem6/1(In1)
  Constant7/1 -> If Action Subsystem5/1(In1)
  Constant8/1 -> If Action Subsystem7/1(In1)
  If Action Subsystem10/1(Out1) -> Merge/8
  If Action Subsystem9/1(Out1) -> Merge/9
  If Action Subsystem8/1(Out1) -> Merge/10
  Demux/3 -> [RS3]
  Demux/2 -> [RS2]
  Demux/1 -> [RS1]
  Demux/7 -> [RS10]
  Demux/8 -> [RS20]
  Demux/9 -> [RS30]
  Demux/10 -> [RS40]
  Demux/11 -> [RS50]
  Demux/12 -> [RS60]
  Demux/6 -> [RS6]
  Demux/5 -> [RS5]
  Demux/4 -> [RS4]
  Constant1/1 -> If Action Subsystem4/1(In1)
  Constant5/1 -> If Action Subsystem/1(In1)
  In1/1 -> Switch Case/1

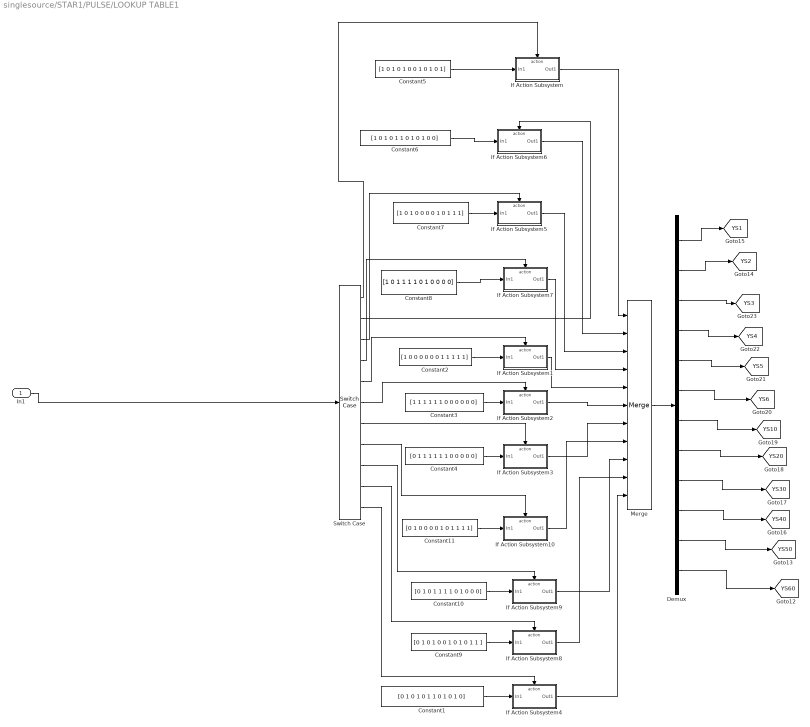
== system singlesource/STAR1/PULSE/LOOKUP TABLE1 ==
  In1 : Inport
  Constant1 : Constant  Value=[0 1 0 1 0 1 1 0 1 0 1 0]
  Constant10 : Constant  Value=[0 1 0 1 1 1 1 0 1 0 0 0]
  Constant11 : Constant  Value=[0 1 0 0 0 0 1 0 1 1 1 1]
  Constant2 : Constant  Value=[1 0 0 0 0 0 0 1 1 1 1 1]
  Constant3 : Constant  Value=[1 1 1 1 1 1 0 0 0 0 0 0]
  Constant4 : Constant  Value=[0 1 1 1 1 1 1 0 0 0 0 0]
  Constant5 : Constant  Value=[1 0 1 0 1 0 0 1 0 1 0 1]
  Constant6 : Constant  Value=[1 0 1 0 1 1 0 1 0 1 0 0]
  Constant7 : Constant  Value=[1 0 1 0 0 0 0 1 0 1 1 1]
  Constant8 : Constant  Value=[1 0 1 1 1 1 0 1 0 0 0 0]
  Constant9 : Constant  Value=[0 1 0 1 0 0 1 0 1 0 1 1 ]
  Demux : Demux  Outputs=12
  If Action Subsystem : Subsystem  TreatAsAtomicUnit=on
  If Action Subsystem1 : Subsystem  TreatAsAtomicUnit=on
  If Action Subsystem10 : Subsystem  TreatAsAtomicUnit=on
  If Action Subsystem2 : Subsystem  TreatAsAtomicUnit=on
  If Action Subsystem3 : Subsystem  TreatAsAtomicUnit=on
  If Action Subsystem4 : Subsystem  TreatAsAtomicUnit=on
  If Action Subsystem5 : Subsystem  TreatAsAtomicUnit=on
  If Action Subsystem6 : Subsystem  TreatAsAtomicUnit=on
  If Action Subsystem7 : Subsystem  TreatAsAtomicUnit=on
  If Action Subsystem8 : Subsystem  TreatAsAtomicUnit=on
  If Action Subsystem9 : Subsystem  TreatAsAtomicUnit=on
  Merge : Merge  Inputs=11
  Switch Case : SwitchCase  CaseConditions={-5 -4 -3 -2 -1 0 1 2 3 4 5}  ShowDefaultCase=off
  tag scope: YS10=global, YS1=global, YS20=global, YS2=global, YS30=global, YS3=global, YS40=global, YS4=global, YS50=global, YS5=global, YS60=global, YS6=global
  wires:
  In1/1 -> Switch Case/1
  Constant5/1 -> If Action Subsystem/1(In1)
  Constant1/1 -> If Action Subsystem4/1(In1)
  If Action Subsystem8/1(Out1) -> Merge/10
  If Action Subsystem9/1(Out1) -> Merge/9
  If Action Subsystem10/1(Out1) -> Merge/8
  Constant8/1 -> If Action Subsystem7/1(In1)
  Constant7/1 -> If Action Subsystem5/1(In1)
  Constant6/1 -> If Action Subsystem6/1(In1)
  Switch Case/1 -> If Action Subsystem/Action
  Switch Case/2 -> If Action Subsystem6/Action
  Switch Case/3 -> If Action Subsystem5/Action
  Switch Case/4 -> If Action Subsystem7/Action
  Switch Case/5 -> If Action Subsystem1/Action
  Switch Case/7 -> If Action Subsystem3/Action
  Switch Case/8 -> If Action Subsystem10/Action
  Switch Case/9 -> If Action Subsystem9/Action
  Switch Case/10 -> If Action Subsystem8/Action
  If Action Subsystem4/1(Out1) -> Merge/11
  Switch Case/11 -> If Action Subsystem4/Action
  Constant11/1 -> If Action Subsystem10/1(In1)
  Constant10/1 -> If Action Subsystem9/1(In1)
  Constant9/1 -> If Action Subsystem8/1(In1)
  If Action Subsystem3/1(Out1) -> Merge/7
  If Action Subsystem2/1(Out1) -> Merge/6
  If Action Subsystem1/1(Out1) -> Merge/5
  If Action Subsystem7/1(Out1) -> Merge/4
  If Action Subsystem5/1(Out1) -> Merge/3
  If Action Subsystem6/1(Out1) -> Merge/2
  Switch Case/6 -> If Action Subsystem2/Action
  Constant2/1 -> If Action Subsystem1/1(In1)
  Constant3/1 -> If Action Subsystem2/1(In1)
  Constant4/1 -> If Action Subsystem3/1(In1)
  If Action Subsystem/1(Out1) -> Merge/1
  Merge/1 -> Demux/1
  Demux/1 -> [YS1]
  Demux/3 -> [YS3]
  Demux/2 -> [YS2]
  Demux/4 -> [YS4]
  Demux/5 -> [YS5]
  Demux/6 -> [YS6]
  Demux/7 -> [YS10]
  Demux/8 -> [YS20]
  Demux/9 -> [YS30]
  Demux/10 -> [YS40]
  Demux/11 -> [YS50]
  Demux/12 -> [YS60]

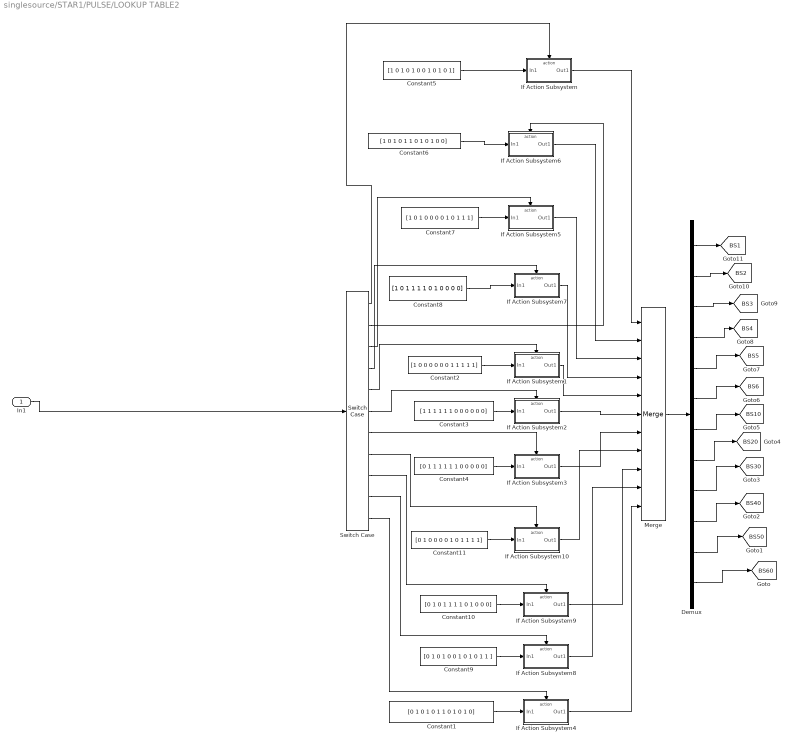
== system singlesource/STAR1/PULSE/LOOKUP TABLE2 ==
  In1 : Inport
  Constant1 : Constant  Value=[0 1 0 1 0 1 1 0 1 0 1 0]
  Constant10 : Constant  Value=[0 1 0 1 1 1 1 0 1 0 0 0]
  Constant11 : Constant  Value=[0 1 0 0 0 0 1 0 1 1 1 1]
  Constant2 : Constant  Value=[1 0 0 0 0 0 0 1 1 1 1 1]
  Constant3 : Constant  Value=[1 1 1 1 1 1 0 0 0 0 0 0]
  Constant4 : Constant  Value=[0 1 1 1 1 1 1 0 0 0 0 0]
  Constant5 : Constant  Value=[1 0 1 0 1 0 0 1 0 1 0 1]
  Constant6 : Constant  Value=[1 0 1 0 1 1 0 1 0 1 0 0]
  Constant7 : Constant  Value=[1 0 1 0 0 0 0 1 0 1 1 1]
  Constant8 : Constant  Value=[1 0 1 1 1 1 0 1 0 0 0 0]
  Constant9 : Constant  Value=[0 1 0 1 0 0 1 0 1 0 1 1 ]
  Demux : Demux  Outputs=12
  If Action Subsystem : Subsystem  TreatAsAtomicUnit=on
  If Action Subsystem1 : Subsystem  TreatAsAtomicUnit=on
  If Action Subsystem10 : Subsystem  TreatAsAtomicUnit=on
  If Action Subsystem2 : Subsystem  TreatAsAtomicUnit=on
  If Action Subsystem3 : Subsystem  TreatAsAtomicUnit=on
  If Action Subsystem4 : Subsystem  TreatAsAtomicUnit=on
  If Action Subsystem5 : Subsystem  TreatAsAtomicUnit=on
  If Action Subsystem6 : Subsystem  TreatAsAtomicUnit=on
  If Action Subsystem7 : Subsystem  TreatAsAtomicUnit=on
  If Action Subsystem8 : Subsystem  TreatAsAtomicUnit=on
  If Action Subsystem9 : Subsystem  TreatAsAtomicUnit=on
  Merge : Merge  Inputs=11
  Switch Case : SwitchCase  CaseConditions={-5 -4 -3 -2 -1 0 1 2 3 4 5}  ShowDefaultCase=off
  tag scope: BS10=global, BS1=global, BS20=global, BS2=global, BS30=global, BS3=global, BS40=global, BS4=global, BS50=global, BS5=global, BS60=global, BS6=global
  wires:
  Merge/1 -> Demux/1
  If Action Subsystem/1(Out1) -> Merge/1
  Constant4/1 -> If Action Subsystem3/1(In1)
  Constant3/1 -> If Action Subsystem2/1(In1)
  Constant2/1 -> If Action Subsystem1/1(In1)
  Switch Case/6 -> If Action Subsystem2/Action
  If Action Subsystem6/1(Out1) -> Merge/2
  If Action Subsystem5/1(Out1) -> Merge/3
  If Action Subsystem7/1(Out1) -> Merge/4
  If Action Subsystem1/1(Out1) -> Merge/5
  If Action Subsystem2/1(Out1) -> Merge/6
  If Action Subsystem3/1(Out1) -> Merge/7
  Constant9/1 -> If Action Subsystem8/1(In1)
  Constant10/1 -> If Action Subsystem9/1(In1)
  Constant11/1 -> If Action Subsystem10/1(In1)
  Switch Case/11 -> If Action Subsystem4/Action
  If Action Subsystem4/1(Out1) -> Merge/11
  Switch Case/10 -> If Action Subsystem8/Action
  Switch Case/9 -> If Action Subsystem9/Action
  Switch Case/8 -> If Action Subsystem10/Action
  Switch Case/7 -> If Action Subsystem3/Action
  Switch Case/5 -> If Action Subsystem1/Action
  Switch Case/4 -> If Action Subsystem7/Action
  Switch Case/3 -> If Action Subsystem5/Action
  Switch Case/2 -> If Action Subsystem6/Action
  Switch Case/1 -> If Action Subsystem/Action
  Constant6/1 -> If Action Subsystem6/1(In1)
  Constant7/1 -> If Action Subsystem5/1(In1)
  Constant8/1 -> If Action Subsystem7/1(In1)
  If Action Subsystem10/1(Out1) -> Merge/8
  If Action Subsystem9/1(Out1) -> Merge/9
  If Action Subsystem8/1(Out1) -> Merge/10
  Constant1/1 -> If Action Subsystem4/1(In1)
  Constant5/1 -> If Action Subsystem/1(In1)
  In1/1 -> Switch Case/1
  Demux/1 -> [BS1]
  Demux/2 -> [BS2]
  Demux/3 -> [BS3]
  Demux/4 -> [BS4]
  Demux/6 -> [BS6]
  Demux/5 -> [BS5]
  Demux/7 -> [BS10]
  Demux/8 -> [BS20]
  Demux/11 -> [BS50]
  Demux/10 -> [BS40]
  Demux/9 -> [BS30]
  Demux/12 -> [BS60]

== system singlesource/STAR1/PULSE/R1 ==
  Product : Product
  Signal Builder : Subsystem  Tag=STV Subsys  LoadFcn=sigbuilder_block('load');  StartFcn=sigbuilder_block('start');  StopFcn=sigbuilder_block('stop');  ClipboardFcn=sigbuilder_block('clipboard');  mask(Sigbuilder block){}
      mask help: Simulink:masks:SigbuilderBlock_MD
      mask init:
      | if ~strcmp(get_param(bdroot(gcbh),'SimulationStatus'),'stopped') tuvar = sigbuilder_block('maskInit'); end
      settings: CopyFcn=sigbuilder_block('copy');  DeleteFcn=sigbuilder_block('delete');  ModelCloseFcn=sigbuilder_block('modelClose');  PreSaveFcn=sigbuilder_block('preSave');  PauseFcn=sigbuilder_block('pause');  ContinueFcn=sigbuilder_block('continue');  NameChangeFcn=sigbuilder_block('namechange');  OpenFcn=sigbuilder_block('open',[437.6 199.2 550.4 400 ]);  CloseFcn=sigbuilder_block('close');
      mask Display: plot(0, 0, 100, 100,[2, 2, 32, 32, 2], [68, 8, 8, 68, 68],[32, 2], [38, 38], [32, 19, 2],[53, 60, 44], [32, 17, 17, 2],[16, 16, 31, 31]);txt = getActiveGroup(gcbh);text(2, 100, txt,'verticalAlignment', 'top');
  Sine Wave : Sin  Amplitude=5*m  Frequency=2*pi*50  SampleTime=0
  Out1 : Outport
  wires:
  Sine Wave/1 -> Out1/1, Product/1
  Signal Builder/1(Signal 1) -> Product/2

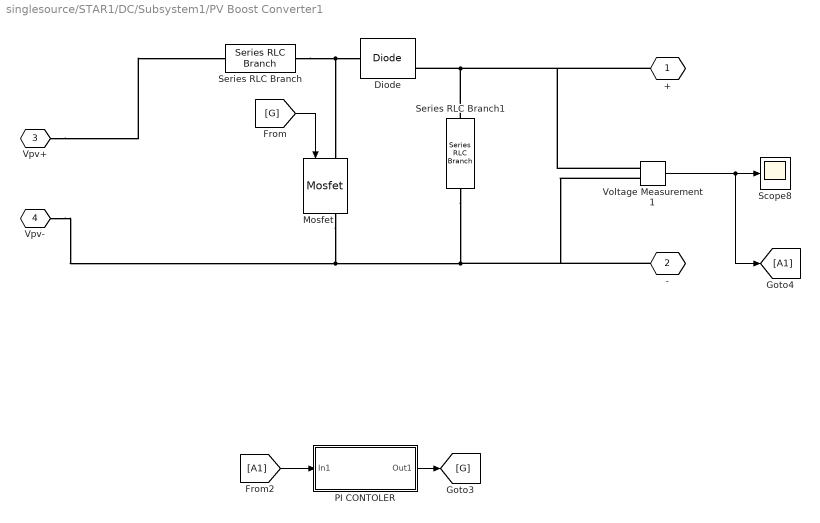
== system singlesource/STAR1/DC/Subsystem1/PV Boost Converter1 ==
  Diode : powerlib/Power Electronics/Diode  Ron=0.001  Lon=0  Vf=0.8  IC=0  UseSnubber=off  Rs=500  Cs=250e-9  Measurements=on
  Mosfet : powerlib/Power Electronics/Mosfet  Ron=0.1  Lon=0  Rd=0.01  Vfd=0  IC=0  Rs=1e5  Cs=inf  Measurements=on
  PI CONTOLER : Subsystem
  Scope8 : Scope
      settings: YMin=66.25  YMax=66.75  SaveName=ScopeData4
  Series RLC Branch : powerlib/Elements/Series RLC Branch  LConnTagsString=__new0  RConnTagsString=__new0  BranchType=L  Resistance=1  Inductance=1e-3  SetiL0=off  InitialCurrent=0  Capacitance=1e-6  Setx0=off  InitialVoltage=0  Measurements=None
  Series RLC Branch1 : powerlib/Elements/Series RLC Branch  LConnTagsString=__new0  RConnTagsString=__new0  BranchType=C  Resistance=1  Inductance=12e-3  SetiL0=off  InitialCurrent=0  Capacitance=1000e-6  Setx0=off  InitialVoltage=0  Measurements=None
  Voltage Measurement1 : powerlib/Measurements/Voltage Measurement  PhasorSimulation=off  OutputType=Complex  PSBequivalent=0
  + : PMIOPort  Port=1  Side=Right
  - : PMIOPort  Port=2  Side=Right
  Vpv+ : PMIOPort  Tag=PMCPort  Port=3  Side=Left
  Vpv- : PMIOPort  Tag=PMCPort  Port=4  Side=Left
  wires:
  [G] -> Mosfet/1
  PI CONTOLER/1(Out1) -> [G]
  [A1] -> PI CONTOLER/1(In1)
  Voltage Measurement1/1 -> [A1], Scope8/1
  connections:
  Series RLC Branch/RConn1 -- Mosfet/LConn1 -- Diode/LConn1
  Mosfet/RConn1 -- Vpv-/RConn1 -- Series RLC Branch1/RConn1 -- -/RConn1 -- Voltage Measurement1/LConn2
  Vpv+/RConn1 -- Series RLC Branch/LConn1
  Series RLC Branch1/LConn1 -- Diode/RConn1 -- +/RConn1 -- Voltage Measurement1/LConn1

== system singlesource/STAR1/DC/Subsystem2/PV Boost Converter1 ==
  Diode : powerlib/Power Electronics/Diode  Ron=0.001  Lon=0  Vf=0.8  IC=0  UseSnubber=off  Rs=500  Cs=250e-9  Measurements=on
  Mosfet : powerlib/Power Electronics/Mosfet  Ron=0.1  Lon=0  Rd=0.01  Vfd=0  IC=0  Rs=1e5  Cs=inf  Measurements=on
  PI CONTOLER : Subsystem
  Scope8 : Scope
      settings: YMin=66.25  YMax=66.75  SaveName=ScopeData4
  Series RLC Branch : powerlib/Elements/Series RLC Branch  LConnTagsString=__new0  RConnTagsString=__new0  BranchType=L  Resistance=1  Inductance=1e-3  SetiL0=off  InitialCurrent=0  Capacitance=1e-6  Setx0=off  InitialVoltage=0  Measurements=None
  Series RLC Branch1 : powerlib/Elements/Series RLC Branch  LConnTagsString=__new0  RConnTagsString=__new0  BranchType=C  Resistance=1  Inductance=12e-3  SetiL0=off  InitialCurrent=0  Capacitance=1000e-6  Setx0=off  InitialVoltage=0  Measurements=None
  Voltage Measurement1 : powerlib/Measurements/Voltage Measurement  PhasorSimulation=off  OutputType=Complex  PSBequivalent=0
  + : PMIOPort  Port=1  Side=Right
  - : PMIOPort  Port=2  Side=Right
  Vpv+ : PMIOPort  Tag=PMCPort  Port=3  Side=Left
  Vpv- : PMIOPort  Tag=PMCPort  Port=4  Side=Left
  wires:
  Voltage Measurement1/1 -> Scope8/1, [A1]
  [A1] -> PI CONTOLER/1(In1)
  PI CONTOLER/1(Out1) -> [G]
  [G] -> Mosfet/1
  connections:
  Voltage Measurement1/LConn1 -- +/RConn1 -- Diode/RConn1 -- Series RLC Branch1/LConn1
  Vpv+/RConn1 -- Series RLC Branch/LConn1
  Voltage Measurement1/LConn2 -- -/RConn1 -- Series RLC Branch1/RConn1 -- Vpv-/RConn1 -- Mosfet/RConn1
  Diode/LConn1 -- Mosfet/LConn1 -- Series RLC Branch/RConn1

== system singlesource/STAR1/DC/Subsystem3/PV Boost Converter1 ==
  Diode : powerlib/Power Electronics/Diode  Ron=0.001  Lon=0  Vf=0.8  IC=0  UseSnubber=off  Rs=500  Cs=250e-9  Measurements=on
  Mosfet : powerlib/Power Electronics/Mosfet  Ron=0.1  Lon=0  Rd=0.01  Vfd=0  IC=0  Rs=1e5  Cs=inf  Measurements=on
  PI CONTOLER : Subsystem
  Scope8 : Scope
      settings: YMin=66.25  YMax=66.75  SaveName=ScopeData4
  Series RLC Branch : powerlib/Elements/Series RLC Branch  LConnTagsString=__new0  RConnTagsString=__new0  BranchType=L  Resistance=1  Inductance=1e-3  SetiL0=off  InitialCurrent=0  Capacitance=1e-6  Setx0=off  InitialVoltage=0  Measurements=None
  Series RLC Branch1 : powerlib/Elements/Series RLC Branch  LConnTagsString=__new0  RConnTagsString=__new0  BranchType=C  Resistance=1  Inductance=12e-3  SetiL0=off  InitialCurrent=0  Capacitance=1000e-6  Setx0=off  InitialVoltage=0  Measurements=None
  Voltage Measurement1 : powerlib/Measurements/Voltage Measurement  PhasorSimulation=off  OutputType=Complex  PSBequivalent=0
  + : PMIOPort  Port=1  Side=Right
  - : PMIOPort  Port=2  Side=Right
  Vpv+ : PMIOPort  Tag=PMCPort  Port=3  Side=Left
  Vpv- : PMIOPort  Tag=PMCPort  Port=4  Side=Left
  wires:
  Voltage Measurement1/1 -> Scope8/1, [A1]
  [A1] -> PI CONTOLER/1(In1)
  PI CONTOLER/1(Out1) -> [G]
  [G] -> Mosfet/1
  connections:
  Voltage Measurement1/LConn1 -- +/RConn1 -- Diode/RConn1 -- Series RLC Branch1/LConn1
  Vpv+/RConn1 -- Series RLC Branch/LConn1
  Voltage Measurement1/LConn2 -- -/RConn1 -- Series RLC Branch1/RConn1 -- Vpv-/RConn1 -- Mosfet/RConn1
  Diode/LConn1 -- Mosfet/LConn1 -- Series RLC Branch/RConn1

== system singlesource/STAR1/DC/Subsystem4/PV Boost Converter1 ==
  Diode : powerlib/Power Electronics/Diode  Ron=0.001  Lon=0  Vf=0.8  IC=0  UseSnubber=off  Rs=500  Cs=250e-9  Measurements=on
  Mosfet : powerlib/Power Electronics/Mosfet  Ron=0.1  Lon=0  Rd=0.01  Vfd=0  IC=0  Rs=1e5  Cs=inf  Measurements=on
  PI CONTOLER : Subsystem
  Scope8 : Scope
      settings: YMin=66.25  YMax=66.75  SaveName=ScopeData4
  Series RLC Branch : powerlib/Elements/Series RLC Branch  LConnTagsString=__new0  RConnTagsString=__new0  BranchType=L  Resistance=1  Inductance=1e-3  SetiL0=off  InitialCurrent=0  Capacitance=1e-6  Setx0=off  InitialVoltage=0  Measurements=None
  Series RLC Branch1 : powerlib/Elements/Series RLC Branch  LConnTagsString=__new0  RConnTagsString=__new0  BranchType=C  Resistance=1  Inductance=12e-3  SetiL0=off  InitialCurrent=0  Capacitance=1000e-6  Setx0=off  InitialVoltage=0  Measurements=None
  Voltage Measurement1 : powerlib/Measurements/Voltage Measurement  PhasorSimulation=off  OutputType=Complex  PSBequivalent=0
  + : PMIOPort  Port=1  Side=Right
  - : PMIOPort  Port=2  Side=Right
  Vpv+ : PMIOPort  Tag=PMCPort  Port=3  Side=Left
  Vpv- : PMIOPort  Tag=PMCPort  Port=4  Side=Left
  wires:
  [G] -> Mosfet/1
  PI CONTOLER/1(Out1) -> [G]
  [A1] -> PI CONTOLER/1(In1)
  Voltage Measurement1/1 -> [A1], Scope8/1
  connections:
  Series RLC Branch/RConn1 -- Mosfet/LConn1 -- Diode/LConn1
  Mosfet/RConn1 -- Vpv-/RConn1 -- Series RLC Branch1/RConn1 -- -/RConn1 -- Voltage Measurement1/LConn2
  Vpv+/RConn1 -- Series RLC Branch/LConn1
  Series RLC Branch1/LConn1 -- Diode/RConn1 -- +/RConn1 -- Voltage Measurement1/LConn1

== system singlesource/STAR1/DC/Subsystem6/PV Boost Converter1 ==
  Diode : powerlib/Power Electronics/Diode  Ron=0.001  Lon=0  Vf=0.8  IC=0  UseSnubber=off  Rs=500  Cs=250e-9  Measurements=on
  Mosfet : powerlib/Power Electronics/Mosfet  Ron=0.1  Lon=0  Rd=0.01  Vfd=0  IC=0  Rs=1e5  Cs=inf  Measurements=on
  PI CONTOLER : Subsystem
  Scope8 : Scope
      settings: YMin=66.25  YMax=66.75  SaveName=ScopeData4
  Series RLC Branch : powerlib/Elements/Series RLC Branch  LConnTagsString=__new0  RConnTagsString=__new0  BranchType=L  Resistance=1  Inductance=1e-3  SetiL0=off  InitialCurrent=0  Capacitance=1e-6  Setx0=off  InitialVoltage=0  Measurements=None
  Series RLC Branch1 : powerlib/Elements/Series RLC Branch  LConnTagsString=__new0  RConnTagsString=__new0  BranchType=C  Resistance=1  Inductance=12e-3  SetiL0=off  InitialCurrent=0  Capacitance=1000e-6  Setx0=off  InitialVoltage=0  Measurements=None
  Voltage Measurement1 : powerlib/Measurements/Voltage Measurement  PhasorSimulation=off  OutputType=Complex  PSBequivalent=0
  + : PMIOPort  Port=1  Side=Right
  - : PMIOPort  Port=2  Side=Right
  Vpv+ : PMIOPort  Tag=PMCPort  Port=3  Side=Left
  Vpv- : PMIOPort  Tag=PMCPort  Port=4  Side=Left
  wires:
  Voltage Measurement1/1 -> Scope8/1, [A1]
  [A1] -> PI CONTOLER/1(In1)
  PI CONTOLER/1(Out1) -> [G]
  [G] -> Mosfet/1
  connections:
  Voltage Measurement1/LConn1 -- +/RConn1 -- Diode/RConn1 -- Series RLC Branch1/LConn1
  Vpv+/RConn1 -- Series RLC Branch/LConn1
  Voltage Measurement1/LConn2 -- -/RConn1 -- Series RLC Branch1/RConn1 -- Vpv-/RConn1 -- Mosfet/RConn1
  Diode/LConn1 -- Mosfet/LConn1 -- Series RLC Branch/RConn1

== system singlesource/STAR1/DC1/Subsystem1/PV Boost Converter1 ==
  Diode : powerlib/Power Electronics/Diode  Ron=0.001  Lon=0  Vf=0.8  IC=0  UseSnubber=off  Rs=500  Cs=250e-9  Measurements=on
  Mosfet : powerlib/Power Electronics/Mosfet  Ron=0.1  Lon=0  Rd=0.01  Vfd=0  IC=0  Rs=1e5  Cs=inf  Measurements=on
  PI CONTOLER : Subsystem
  Scope8 : Scope
      settings: YMin=66.25  YMax=66.75  SaveName=ScopeData4
  Series RLC Branch : powerlib/Elements/Series RLC Branch  LConnTagsString=__new0  RConnTagsString=__new0  BranchType=L  Resistance=1  Inductance=1e-3  SetiL0=off  InitialCurrent=0  Capacitance=1e-6  Setx0=off  InitialVoltage=0  Measurements=None
  Series RLC Branch1 : powerlib/Elements/Series RLC Branch  LConnTagsString=__new0  RConnTagsString=__new0  BranchType=C  Resistance=1  Inductance=12e-3  SetiL0=off  InitialCurrent=0  Capacitance=1000e-6  Setx0=off  InitialVoltage=0  Measurements=None
  Voltage Measurement1 : powerlib/Measurements/Voltage Measurement  PhasorSimulation=off  OutputType=Complex  PSBequivalent=0
  + : PMIOPort  Port=1  Side=Right
  - : PMIOPort  Port=2  Side=Right
  Vpv+ : PMIOPort  Tag=PMCPort  Port=3  Side=Left
  Vpv- : PMIOPort  Tag=PMCPort  Port=4  Side=Left
  wires:
  Voltage Measurement1/1 -> Scope8/1, [A1]
  [A1] -> PI CONTOLER/1(In1)
  PI CONTOLER/1(Out1) -> [G]
  [G] -> Mosfet/1
  connections:
  Voltage Measurement1/LConn1 -- +/RConn1 -- Diode/RConn1 -- Series RLC Branch1/LConn1
  Vpv+/RConn1 -- Series RLC Branch/LConn1
  Voltage Measurement1/LConn2 -- -/RConn1 -- Series RLC Branch1/RConn1 -- Vpv-/RConn1 -- Mosfet/RConn1
  Diode/LConn1 -- Mosfet/LConn1 -- Series RLC Branch/RConn1

== system singlesource/STAR1/DC1/Subsystem2/PV Boost Converter1 ==
  Diode : powerlib/Power Electronics/Diode  Ron=0.001  Lon=0  Vf=0.8  IC=0  UseSnubber=off  Rs=500  Cs=250e-9  Measurements=on
  Mosfet : powerlib/Power Electronics/Mosfet  Ron=0.1  Lon=0  Rd=0.01  Vfd=0  IC=0  Rs=1e5  Cs=inf  Measurements=on
  PI CONTOLER : Subsystem
  Scope8 : Scope
      settings: YMin=66.25  YMax=66.75  SaveName=ScopeData4
  Series RLC Branch : powerlib/Elements/Series RLC Branch  LConnTagsString=__new0  RConnTagsString=__new0  BranchType=L  Resistance=1  Inductance=1e-3  SetiL0=off  InitialCurrent=0  Capacitance=1e-6  Setx0=off  InitialVoltage=0  Measurements=None
  Series RLC Branch1 : powerlib/Elements/Series RLC Branch  LConnTagsString=__new0  RConnTagsString=__new0  BranchType=C  Resistance=1  Inductance=12e-3  SetiL0=off  InitialCurrent=0  Capacitance=1000e-6  Setx0=off  InitialVoltage=0  Measurements=None
  Voltage Measurement1 : powerlib/Measurements/Voltage Measurement  PhasorSimulation=off  OutputType=Complex  PSBequivalent=0
  + : PMIOPort  Port=1  Side=Right
  - : PMIOPort  Port=2  Side=Right
  Vpv+ : PMIOPort  Tag=PMCPort  Port=3  Side=Left
  Vpv- : PMIOPort  Tag=PMCPort  Port=4  Side=Left
  wires:
  [G] -> Mosfet/1
  PI CONTOLER/1(Out1) -> [G]
  [A1] -> PI CONTOLER/1(In1)
  Voltage Measurement1/1 -> [A1], Scope8/1
  connections:
  Series RLC Branch/RConn1 -- Mosfet/LConn1 -- Diode/LConn1
  Mosfet/RConn1 -- Vpv-/RConn1 -- Series RLC Branch1/RConn1 -- -/RConn1 -- Voltage Measurement1/LConn2
  Vpv+/RConn1 -- Series RLC Branch/LConn1
  Series RLC Branch1/LConn1 -- Diode/RConn1 -- +/RConn1 -- Voltage Measurement1/LConn1

== system singlesource/STAR1/DC1/Subsystem3/PV Boost Converter1 ==
  Diode : powerlib/Power Electronics/Diode  Ron=0.001  Lon=0  Vf=0.8  IC=0  UseSnubber=off  Rs=500  Cs=250e-9  Measurements=on
  Mosfet : powerlib/Power Electronics/Mosfet  Ron=0.1  Lon=0  Rd=0.01  Vfd=0  IC=0  Rs=1e5  Cs=inf  Measurements=on
  PI CONTOLER : Subsystem
  Scope8 : Scope
      settings: YMin=66.25  YMax=66.75  SaveName=ScopeData4
  Series RLC Branch : powerlib/Elements/Series RLC Branch  LConnTagsString=__new0  RConnTagsString=__new0  BranchType=L  Resistance=1  Inductance=1e-3  SetiL0=off  InitialCurrent=0  Capacitance=1e-6  Setx0=off  InitialVoltage=0  Measurements=None
  Series RLC Branch1 : powerlib/Elements/Series RLC Branch  LConnTagsString=__new0  RConnTagsString=__new0  BranchType=C  Resistance=1  Inductance=12e-3  SetiL0=off  InitialCurrent=0  Capacitance=1000e-6  Setx0=off  InitialVoltage=0  Measurements=None
  Voltage Measurement1 : powerlib/Measurements/Voltage Measurement  PhasorSimulation=off  OutputType=Complex  PSBequivalent=0
  + : PMIOPort  Port=1  Side=Right
  - : PMIOPort  Port=2  Side=Right
  Vpv+ : PMIOPort  Tag=PMCPort  Port=3  Side=Left
  Vpv- : PMIOPort  Tag=PMCPort  Port=4  Side=Left
  wires:
  [G] -> Mosfet/1
  PI CONTOLER/1(Out1) -> [G]
  [A1] -> PI CONTOLER/1(In1)
  Voltage Measurement1/1 -> [A1], Scope8/1
  connections:
  Series RLC Branch/RConn1 -- Mosfet/LConn1 -- Diode/LConn1
  Mosfet/RConn1 -- Vpv-/RConn1 -- Series RLC Branch1/RConn1 -- -/RConn1 -- Voltage Measurement1/LConn2
  Vpv+/RConn1 -- Series RLC Branch/LConn1
  Series RLC Branch1/LConn1 -- Diode/RConn1 -- +/RConn1 -- Voltage Measurement1/LConn1
